simulink model "sliding mode control"  (R2022a)
settings: Solver=VariableStepAuto  StartTime=0.0  StopTime=20  RelTol=1e-3
libraries: simulink x1
settings Model: Creator=Yu  LastModifiedBy=Yu

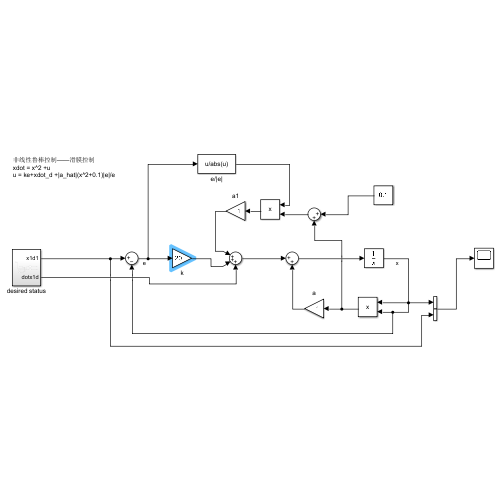
[thumbnail: Simulink's stored preview of the top-level diagram]
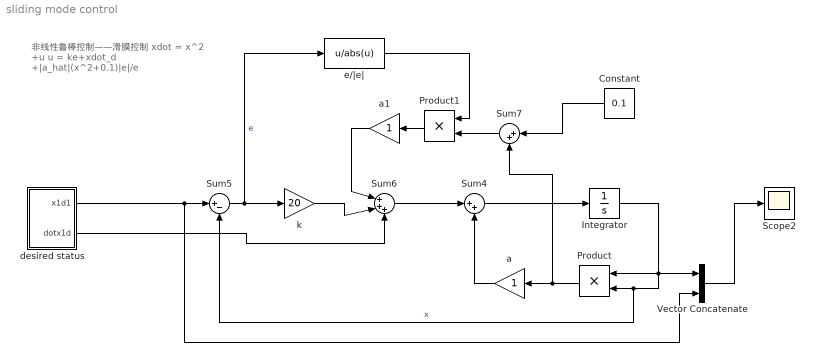
== system sliding mode control ==
  note: 非线性鲁棒控制——滑膜控制
      | xdot = x^2 +u
      | u = ke+xdot_d +|a_hat|(x^2+0.1)|e|/e
  Constant : Constant  Value=0.1
  Integrator : Integrator
  Product : Product
  Product1 : Product
  Scope2 : Scope
  Sum4 : Sum  Inputs=|++
  Sum5 : Sum  Inputs=|+-
  Sum6 : Sum  Inputs=|+++
  Sum7 : Sum  Inputs=|++
  Vector Concatenate : Concatenate
  a : Gain
  a1 : Gain
  desired status : Subsystem
  e/|e| : Fcn  Expr=u/abs(u)
  k : Gain  Gain=20
  wires:
  Integrator/1 -> Vector Concatenate/1, Sum5/2, Product/2, Product/1  "x"
  Product/1 -> Sum7/2, a/1
  a/1 -> Sum4/2
  Sum4/1 -> Integrator/1
  Sum5/1 -> e/|e|/1, k/1  "e"
  desired status/1(x1d1) -> Vector Concatenate/2, Sum5/1
  desired status/2(dotx1d) -> Sum6/3
  k/1 -> Sum6/2
  Sum6/1 -> Sum4/1
  Constant/1 -> Sum7/1
  Sum7/1 -> Product1/2
  e/|e|/1 -> Product1/1
  Product1/1 -> a1/1
  a1/1 -> Sum6/1
  Vector Concatenate/1 -> Scope2/1

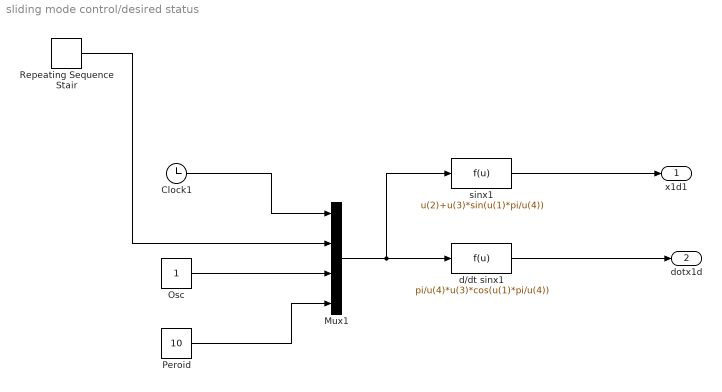
== system sliding mode control/desired status ==
  Clock1 : Clock
      settings: Decimation=100
  Mux1 : Mux
  Osc : Constant
  Peroid : Constant  Value=10
  Repeating Sequence Stair : simulink/Sources/Repeating Sequence Stair  OutValues=[1 0 1 0 1].'  tsamp=10  OutMin=[]  OutMax=[]  OutDataTypeStr=double  OutputDataTypeScalingMode=double  OutDataType=fixdt(0,8)  ConRadixGroup=Best Precision: Vector-wise  OutScaling=2^-12
  d/dt sinx1 : Fcn  Expr=pi/u(4)*u(3)*cos(u(1)*pi/u(4))
  sinx1 : Fcn  Expr=u(2)+u(3)*sin(u(1)*pi/u(4))
  x1d1 : Outport
  dotx1d : Outport  Port=2
  wires:
  Mux1/1 -> sinx1/1, d/dt sinx1/1
  Repeating Sequence Stair/1 -> Mux1/2
  sinx1/1 -> x1d1/1
  Clock1/1 -> Mux1/1
  Peroid/1 -> Mux1/4
  d/dt sinx1/1 -> dotx1d/1
  Osc/1 -> Mux1/3
